simulink model "MSRI-Up_Code"  (R2024b)
settings: Solver=ode15s  StartTime=0.0  StopTime=5000  RelTol=1e-6  AbsTol=1e-6  EnableMultiTasking=on
settings Model: Creator=Usuario  LastModifiedBy=russj
settings SolverCC: DateTimeAtSimulationTimeZero=[]  AutoScaleAbsTol=off  AlgebraicLoopSolver=TrustRegion
settings DataIOCC: LimitDataPoints=on  SaveFormat=Array  ReturnWorkspaceOutputs=off
settings OptimizationCC: LifeSpan=inf
settings DebuggingCC: SolverPrmCheckMsg=warning  UnconnectedInputMsg=warning  UnconnectedOutputMsg=warning  UnconnectedLineMsg=warning  SFUnexpectedBacktrackingDiag=warning  SFNoUnconditionalDefaultTransitionDiag=warning  SFExecutionAtInitializationDiag=none  ArithmeticOperatorsInVariantConditions=warning
settings HardwareCC: ProdBitPerPointer=32  ProdBitPerSizeT=32  ProdBitPerPtrDiffT=32  ProdLargestAtomicFloat=None  ProdIntDivRoundTo=Undefined  ProdEndianess=Unspecified  ProdWordSize=32  ProdHWDeviceType=32-bit Generic
settings ModelReferenceCC: EnableRefExpFcnMdlSchedulingChecks=on  PropagateSignalLabelsOutOfModel=off
settings SFSimCC: SimUseLocalCustomCode=off  CustomCodeUndefinedFunction=UseInterfaceOnly
settings RTWCC: RTWUseLocalCustomCode=off  GPUComputeCapability=3.5  DLArmComputeVersion=19.05
settings CodeAppCC: StateflowObjectComments=on
settings GRTTargetCC: TargetLangStandard=C89/C90 (ANSI)
settings ConfigComp: CovMetricSettings=dw  CovSaveCumulativeToWorkspaceVar=on  CovSaveSingleToWorkspaceVar=on  CovExternalEMLEnable=off  CovSFcnEnable=off

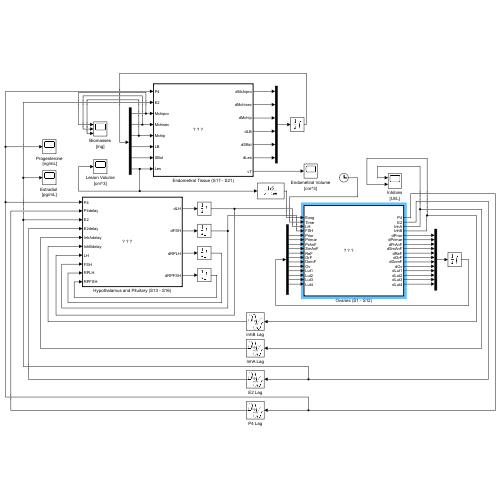
[thumbnail: Simulink's stored preview of the top-level diagram]
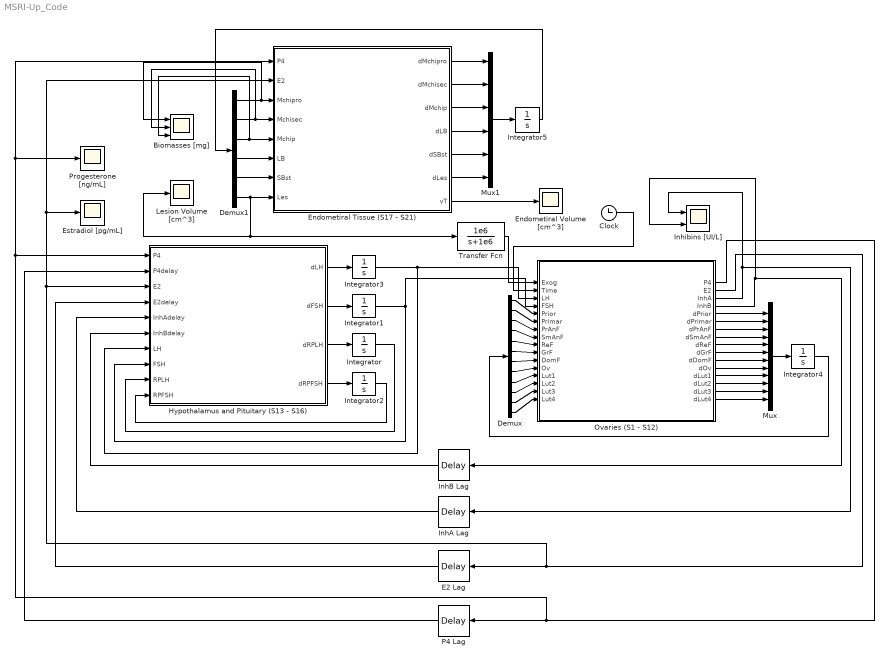
== system MSRI-Up_Code ==
  Biomasses [mg] : Scope  NumInputPorts=3
  Clock : Clock
  Demux : Demux  Outputs=12
  Demux1 : Demux  Outputs=6
  E2 Lag : TransportDelay  DelayTime=0.187
  Endometiral Tissue (S17 - S21) : MATLAB Function  TreatAsAtomicUnit=on
  Endometiral Volume [cm^3] : Scope
  Estradiol [pg/mL] : Scope
  Hypothalamus and Pituitary (S13 - S16) : MATLAB Function  TreatAsAtomicUnit=on
  InhA Lag : TransportDelay  DelayTime=1.38
  InhB Lag : TransportDelay  DelayTime=0
  Inhibins [UI/L] : Scope  NumInputPorts=2
  Integrator : Integrator  InitialCondition=78.5  LimitOutput=on  LowerSaturationLimit=0
  Integrator1 : Integrator  InitialCondition=11  LimitOutput=on  LowerSaturationLimit=0
  Integrator2 : Integrator  InitialCondition=12  LimitOutput=on  LowerSaturationLimit=0
  Integrator3 : Integrator  InitialCondition=9.05  LimitOutput=on  LowerSaturationLimit=0
  Integrator4 : Integrator  InitialCondition=[265000, 100, 1.15, 3.98, 40.4, 53.1, 23.3, 16.0, 91.3, 320, 438, 362]  LimitOutput=on  LowerSaturationLimit=0
  Integrator5 : Integrator  InitialCondition=[1400, 3000, 20, 1, 0, 0.01]  LimitOutput=on  LowerSaturationLimit=0
  Lesion Volume [cm^3] : Scope
  Mux : Mux  Inputs=12
  Mux1 : Mux  Inputs=6
  Ovaries (S1 - S12) : MATLAB Function  TreatAsAtomicUnit=on
  P4 Lag : TransportDelay  DelayTime=2
  Progesterone [ng/mL] : Scope
  Transfer Fcn : TransferFcn  Numerator=[1e6]  Denominator=[1 1e6]
  wires:
  Integrator/1 -> Hypothalamus and Pituitary (S13 - S16)/9(RPLH)
  Integrator3/1 -> Hypothalamus and Pituitary (S13 - S16)/7(LH), Ovaries (S1 - S12)/3(LH)
  Integrator2/1 -> Hypothalamus and Pituitary (S13 - S16)/10(RPFSH)
  Integrator1/1 -> Hypothalamus and Pituitary (S13 - S16)/8(FSH), Ovaries (S1 - S12)/4(FSH)
  Mux/1 -> Integrator4/1
  Ovaries (S1 - S12)/3(InhA) -> Inhibins [UI/L]/1, InhA Lag/1
  InhA Lag/1 -> Hypothalamus and Pituitary (S13 - S16)/5(InhAdelay)
  Hypothalamus and Pituitary (S13 - S16)/1(dLH) -> Integrator3/1
  Hypothalamus and Pituitary (S13 - S16)/2(dFSH) -> Integrator1/1
  Hypothalamus and Pituitary (S13 - S16)/4(dRPFSH) -> Integrator2/1
  Hypothalamus and Pituitary (S13 - S16)/3(dRPLH) -> Integrator/1
  Demux/1 -> Ovaries (S1 - S12)/5(Prior)
  Demux/2 -> Ovaries (S1 - S12)/6(Primar)
  Demux/3 -> Ovaries (S1 - S12)/7(PrAnF)
  Demux/4 -> Ovaries (S1 - S12)/8(SmAnF)
  Demux/5 -> Ovaries (S1 - S12)/9(ReF)
  Demux/6 -> Ovaries (S1 - S12)/10(GrF)
  Demux/7 -> Ovaries (S1 - S12)/11(DomF)
  Demux/8 -> Ovaries (S1 - S12)/12(Ov)
  Demux/9 -> Ovaries (S1 - S12)/13(Lut1)
  Demux/10 -> Ovaries (S1 - S12)/14(Lut2)
  Demux/11 -> Ovaries (S1 - S12)/15(Lut3)
  Demux/12 -> Ovaries (S1 - S12)/16(Lut4)
  Ovaries (S1 - S12)/16(dLut4) -> Mux/12
  Ovaries (S1 - S12)/15(dLut3) -> Mux/11
  Ovaries (S1 - S12)/14(dLut2) -> Mux/10
  Ovaries (S1 - S12)/13(dLut1) -> Mux/9
  Ovaries (S1 - S12)/12(dOv) -> Mux/8
  Ovaries (S1 - S12)/11(dDomF) -> Mux/7
  Ovaries (S1 - S12)/10(dGrF) -> Mux/6
  Ovaries (S1 - S12)/9(dReF) -> Mux/5
  Ovaries (S1 - S12)/8(dSmAnF) -> Mux/4
  Ovaries (S1 - S12)/7(dPrAnF) -> Mux/3
  Ovaries (S1 - S12)/6(dPrimar) -> Mux/2
  Ovaries (S1 - S12)/4(InhB) -> Inhibins [UI/L]/2, InhB Lag/1
  InhB Lag/1 -> Hypothalamus and Pituitary (S13 - S16)/6(InhBdelay)
  Ovaries (S1 - S12)/5(dPrior) -> Mux/1
  Ovaries (S1 - S12)/2(E2) -> Estradiol [pg/mL]/1, Endometiral Tissue (S17 - S21)/2(E2), Hypothalamus and Pituitary (S13 - S16)/3(E2), E2 Lag/1
  E2 Lag/1 -> Hypothalamus and Pituitary (S13 - S16)/4(E2delay)
  Ovaries (S1 - S12)/1(P4) -> Endometiral Tissue (S17 - S21)/1(P4), Progesterone [ng/mL]/1, Hypothalamus and Pituitary (S13 - S16)/1(P4), P4 Lag/1
  P4 Lag/1 -> Hypothalamus and Pituitary (S13 - S16)/2(P4delay)
  Integrator4/1 -> Demux/1
  Endometiral Tissue (S17 - S21)/1(dMchipro) -> Mux1/1
  Endometiral Tissue (S17 - S21)/2(dMchisec) -> Mux1/2
  Endometiral Tissue (S17 - S21)/3(dMchip) -> Mux1/3
  Endometiral Tissue (S17 - S21)/4(dLB) -> Mux1/4
  Endometiral Tissue (S17 - S21)/5(dSBst) -> Mux1/5
  Mux1/1 -> Integrator5/1
  Demux1/1 -> Endometiral Tissue (S17 - S21)/3(Mchipro), Biomasses [mg]/1
  Demux1/2 -> Biomasses [mg]/2, Endometiral Tissue (S17 - S21)/4(Mchisec)
  Demux1/3 -> Endometiral Tissue (S17 - S21)/5(Mchip), Biomasses [mg]/3
  Demux1/4 -> Endometiral Tissue (S17 - S21)/6(LB)
  Demux1/5 -> Endometiral Tissue (S17 - S21)/7(SBst)
  Integrator5/1 -> Demux1/1
  Endometiral Tissue (S17 - S21)/7(vT) -> Endometiral Volume [cm^3]/1
  Clock/1 -> Ovaries (S1 - S12)/2(Time)
  Transfer Fcn/1 -> Ovaries (S1 - S12)/1(Exog)
  Endometiral Tissue (S17 - S21)/6(dLes) -> Mux1/6
  Demux1/6 -> Lesion Volume [cm^3]/1, Transfer Fcn/1, Endometiral Tissue (S17 - S21)/8(Les)

== matlab function MSRI-Up_Code/Ovaries (S1 - S12) ==
  data: Exog input; Time input; P4 output; E2 output; InhA output; InhB output; dPrior output; dPrimar output; dPrAnF output; dSmAnF output; LH input; FSH input; Prior input; Primar input; PrAnF input; SmAnF input; ReF input; GrF input; DomF input; Ov input; dReF output; dGrF output; dDomF output; dOv output; Lut1 input; Lut2 input; Lut3 input; Lut4 input; dLut1 output; dLut2 output; dLut3 output; dLut4 output
function [P4,E2,InhA,InhB,dPrior,dPrimar,dPrAnF,dSmAnF,dReF,dGrF,dDomF,dOv,...
    dLut1,dLut2,dLut3,dLut4]= ...
    fcn(Exog, Time, LH,FSH,Prior,Primar,PrAnF,SmAnF,ReF,GrF,DomF,Ov,Lut1,Lut2,Lut3,Lut4)
%% Parameters ============================================================ (Confirmed)
cAMH = 0.226;      % [mL/ng]
cprm = 1.37E-5;    % [1/follicle]
rsurv = 0.014;     % [~]
r1 = 0.00102;      % [1/day]
r2 = 0.00694;      % [1/day]
a1 = 0.0437;       % [ng/(mL*follicle)]
a2 = 0;            % [~]
a3 = 0;            % [~]

vol2 = 0.500;      % [mm^3]
Kmf1 = 9.82;       % [UI/L]
Kmf2 = 10.4;       % [UI/L]
Kmf3 = 5.08;       % [UI/L]
KiAMH = 20.7;      % [ng/mL]
alpha = 29.1;      % [~]
beta = 2.06;       % [~]
gamma = 2.95;      % [~]
delta = 0.999;     % [~]
omega = 0.363;     % [~]
r3 = 0.759;        % [1/day]
r4 = 2.23;         % [L/(day*UI)]
r5 = 1.21;         % [1/day]
c1 = 0.918;        % [1/day]
c2 = 0.0575;       % [(L/IU)^delta/day]
c3 = 0.0241;       % [L/(IU*day)]
c4 = 0.0307;       % [L/(IU*day)]
c5 = 0.198;        % [(L/IU)^gamma/day]
c6 = 0.00519;      % [L/(IU*day)]
c7 = 0.686;        % [day]
k1 = 0.416;        % [1/day]
k2 = 0.405;        % [1/day]   
k3 = 0.551;        % [1/day]
k4 = 0.903;        % [1/day]

e0 = 30;           % [pg/mL]
e1 = 0.04;         % [pg/(mL*mm^3)]
e2 = 0.065;        % [pg/(mL*mm^3)]
e3 = 0.1;          % [pg/(mL*mm^3)]
p0 = 0;            % [ng/(mL*mm^3)]
p1 = 0.0085;       % [ng/(mL*mm^3)]
p2 = 0;            % [ng/(mL*mm^3)]
h0 = 0;            % [IU/mL]
h1 = 0.0035;       % [IU/(mL*mm^3)]
h2 = 0.0021;       % [IU/(mL*mm^3)]
h3 = 0.0021;       % [IU/(mL*mm^3)]
j0 = 15;           % [IU/mL]
j1 = 20.2;         % [pg/(mL*mm^3)]
j2 = 0.0138;       % [pg/(mL*mm^3)]

%% Algebraic Equations =================================================== (Confirmed)
%if 30 <= Time && Time <= 60 || 90 <= Time && Time <= 120
%    Exog = 5;
%else
%    Exog = 0;
%end 

%for Time = 30:1:60
%    Exog = 2;
%end

eL = 0.5;
E2 = e0 + (e1*GrF) + (e2*DomF) + (e3*Lut4) + (eL*Exog);
P4 = p0 + (p1*Lut3) + (p2*Lut4);
InhA = h0 + (h1*DomF) + (h2*Lut2) + (h3*Lut3);
InhB = j0 + (j1*SmAnF) + (j2*Ov);
AMH = (a1*Primar) + (a2*PrAnF) + (a3*SmAnF);

%% Differential Equations ================================================ (Confirmed)
dPrior = -(r1*Prior)/(1 + cprm*Prior + cAMH*AMH);
dPrimar = ((rsurv*r1*Prior)/(1 + cprm*Prior + cAMH*AMH)) - (r2*Primar);
dPrAnF = (vol2*r2*Primar) - ((r3*PrAnF*(FSH^alpha))/((Kmf1^alpha) + (FSH^alpha)));
dSmAnF = ((r3*PrAnF*(FSH^alpha))/((Kmf1^alpha) + (FSH^alpha))) +...
    (((r4*(FSH^beta))/((Kmf2^beta) + (FSH^beta))) - r5)*SmAnF;
dReF = (r5*SmAnF) + (((c1*(FSH^gamma))/((Kmf3^gamma) + (FSH^gamma))) - (c2*(LH^delta)))*ReF;
dGrF = (c2*(LH^delta)*ReF) + (((c3*FSH)/(1 + (AMH/KiAMH))) - (c4*LH))*GrF;
dDomF = (c4*LH*GrF) - (c5*(LH^omega)*DomF);
dOv = (c5*(LH^omega)*DomF) + (c6*LH*Ov) - (c7*Ov);
dLut1 = (c7*Ov) - (k1*Lut1);
dLut2 = (k1*Lut1) - (k2*Lut2);
dLut3 = (k2*Lut2) - (k3*Lut3);
dLut4 = (k3*Lut3) - (k4*Lut4);

== matlab function MSRI-Up_Code/Hypothalamus and Pituitary (S13 - S16) ==
  data: dLH output; dFSH output; P4 input; P4delay input; dRPLH output; dRPFSH output; E2 input; E2delay input; InhAdelay input; InhBdelay input; LH input; FSH input; RPLH input; RPFSH input
function [dLH, dFSH, dRPLH, dRPFSH] = ...
    fcn(P4, P4delay, E2, E2delay, InhAdelay, InhBdelay, LH, FSH, RPLH, RPFSH)
%% Parameters ============================================================ (Confirmed)
V0LH = 343;            % [IU/day]
V1LH = 8110;           % [IU/day]
KmLH = 247;            % [pg/mL]
KiLHP = 155;           % [ng/mL]
kLH = 1.01;            % [1/day]
clLH = 14;             % [1/day]
cLHP = 1.10;           % [mL/ng]
cLHE = 0.00398;        % [mL/ng]
VFSH = 616;            % [IU/day]
KiFSHInhA = 2.58;      % [IU/mL]
KiFSHInhB = 120;       % [pg/mL]
kFSH = 1.04;           % [1/day]
clFSH = 8.21;          % [1/day]
cFSHP = 130;           % [mL/ng]
cFSHE = 0.00525;       % [mL^2/pg^2]
v = 2.5;               % [L]

%% Differential Equations ================================================ (Confirmed)
dRPLH = ((V0LH + ((V1LH*(E2delay^8))/((KmLH^8) + (E2delay^8))))/(1 + (P4delay/KiLHP))) -...
    ((kLH*(1 + cLHP*P4)*RPLH)/(1 + cLHE*E2));

dLH = ((1/v)*((kLH*(1 + cLHP*P4)*RPLH)/(1 + cLHE*E2))) - (clLH*LH);

dRPFSH = (VFSH/(1 + (InhAdelay/KiFSHInhA) + (InhBdelay/KiFSHInhB))) -...
    ((kFSH*(1 + cFSHP*P4)*RPFSH)/(1 + (cFSHE*(E2^2))));

dFSH = ((1/v)*((kFSH*(1 + cFSHP*P4)*RPFSH)/(1 + (cFSHE*(E2^2))))) - (clFSH*FSH);

== matlab function MSRI-Up_Code/Endometiral Tissue (S17 - S21) ==
  data: dMchipro output; dMchisec output; P4 input; dMchip output; dLB output; E2 input; dSBst output; dLes output; vT output; Mchipro input; Mchisec input; Mchip input; LB input; SBst input; Les input
function [dMchipro, dMchisec, dMchip, dLB, dSBst, dLes, vT] = ...
    fcn(P4, E2, Mchipro, Mchisec, Mchip, LB, SBst, Les)
%% Parameters ============================================================ (Confirmed)
kPro = 0.008417;          % [cm^3/(pg*day)]
ksec = 0.154731;          % [cm^3/(ng*day)]
kd = 20;                  % [~]
Ks = 10;                  % [mg]
mP = 0.001;               % [1/day]
Ms = 1.17;                % [~]
YPchisec = 0.1;           % [~]
Ychisecchipro = 0.45;     % [~]
wchisec6 = 0.9;           % [~]
wp6 = 0.1;                % [~]
rhochipro = 1050;         % [mg/cm^3]
rhochisec = 1050;         % [mg/cm^3]
rhochiP = 1400;           % [mg/cm^3]
muB = 0.0035;             % [Pas]
Aau = 0.015;              % [cm^2]
n = 3000;                 % [~]
deltaP = 0.0005;          % [Pa]
k = 0.1;                  % [~]
lambda = 0.9998;          % [~]
v1 = 777600;              % [cm/day]
kPBE = 70;                % [1/day]
kETR = 1;                 % [mL/(day*pg)]
KmPBE = 0.0005;           % [~]
KmETR = 0.0001;           % [~]
KiPBE = 8;                % [ng/mL]
KiETR = 14;               % [ng/mL]

%% Algebraic Equations =================================================== (Confirmed)
mumaxPro = kPro*E2;
mumaxsec = ksec*P4;
mupro = (mumaxPro*Ms)/(Ks + Ms);
musec = (mumaxsec*Ms)/(Ks + Ms);
mdot6 = kd*SBst*((Mchisec/wchisec6) + (Mchip/wp6));
qP = YPchisec*musec + mP;
vdot1 = v1*Aau;
vdot2 = lambda*v1*Aau;
r = k*LB;
Poiseuillevol = (deltaP*pi*r^4)/(8*muB*LB);
vdot5 = SBst*Poiseuillevol*n;
AB = pi*r^2*n;
rPBEmax = kPBE;
rETRmax = kETR*E2;
rPBE = (rPBEmax*(1 - SBst))/(KmPBE + (1 - SBst))*1/(1 + P4/KiPBE);
rETR = (rETRmax*SBst)/(KmETR + SBst)*1/(1 + P4/KiETR);
vT = Mchipro/rhochipro + Mchisec/rhochisec + Mchip/rhochiP;

%% Differential Equations ================================================ (Confirmed)
dMchipro = (mupro*Mchipro) - (musec*Mchipro);
dMchisec = (Ychisecchipro*musec*Mchipro) - (mdot6*wchisec6);
dMchip = (qP*Mchisec) - (mdot6*wp6);
dLB = (vdot1 - vdot2 - vdot5)/AB;
dSBst = rPBE - rETR;

%% Hypothesized Lesion Volume ============================================ (Confirmed)
kg = 0.008417;
LMax=1;
dLes = kg*Les*(1-Les/LMax);
